simulink model "SensorTuner"  (R2024a)
settings: Solver=FixedStepAuto  StartTime=0.0  StopTime=3980  FixedStep=0.02  MinStep=0.1  RelTol=1e-3
values from neighbouring files (symbols this model uses):
  f = 0    [avg_error_f.m]
undefined symbols (not defined in the file or in its folder): dt, tau
settings Model: Creator=Pedro  LastModifiedBy=Pedro

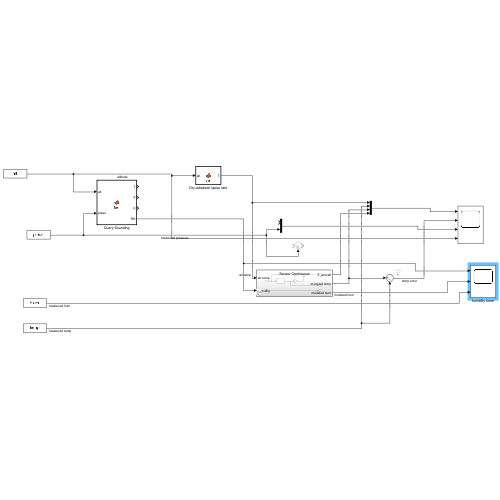
[thumbnail: Simulink's stored preview of the top-level diagram]
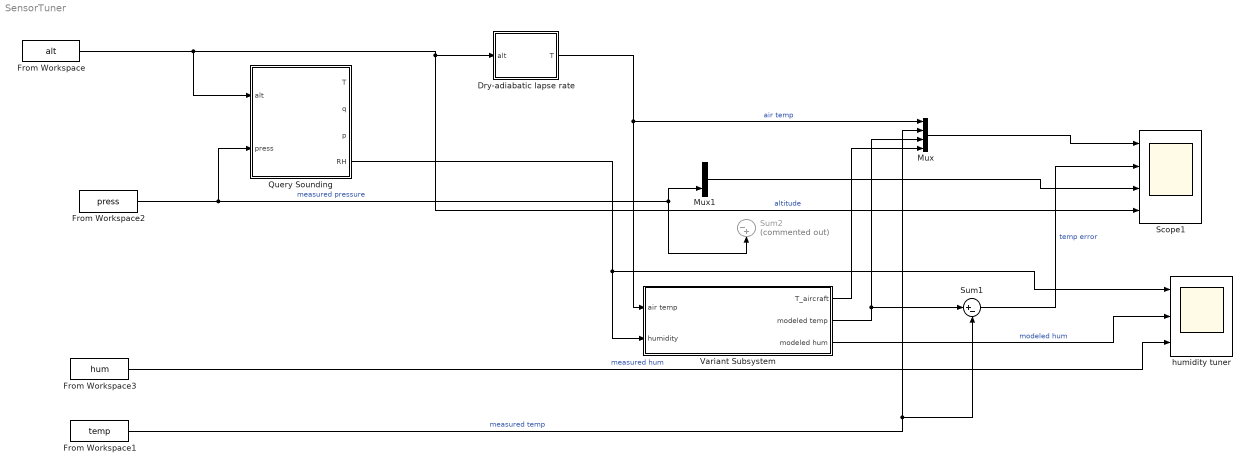
== system SensorTuner ==
  Dry-adiabatic lapse rate : MATLAB Function  TreatAsAtomicUnit=on
  From Workspace : FromWorkspace  VariableName=alt  OutputAfterFinalValue=Setting to zero
  From Workspace1 : FromWorkspace  VariableName=temp
  From Workspace2 : FromWorkspace  VariableName=press
  From Workspace3 : FromWorkspace  VariableName=hum
  Mux : Mux
  Mux1 : Mux  Inputs=2
  Query Sounding : MATLAB Function  TreatAsAtomicUnit=on
  Scope1 : Scope  NumInputPorts=4
  Sum1 : Sum  Inputs=|+-
  Sum2 : Sum  Commented=on  Inputs=|-+
  Variant Subsystem : Subsystem  Variant=on
  humidity tuner : Scope  NumInputPorts=3
  wires:
  Dry-adiabatic lapse rate/1(T) -> Variant Subsystem/1(air temp), Mux/1  "air temp"
  From Workspace/1 -> Query Sounding/1(alt), Dry-adiabatic lapse rate/1(alt), Scope1/4  "altitude"
  Mux/1 -> Scope1/1
  Sum1/1 -> Scope1/2  "temp error"
  From Workspace2/1 -> Query Sounding/2(press), Mux1/2, Sum2/2  "measured pressure"
  Mux1/1 -> Scope1/3
  From Workspace1/1 -> Sum1/2, Mux/2  "measured temp"
  Variant Subsystem/1(T_aircraft) -> Mux/4
  Variant Subsystem/2(modeled temp) -> Mux/3, Sum1/1
  Query Sounding/4(RH) -> humidity tuner/1, Variant Subsystem/2(humidity)
  Variant Subsystem/3(modeled hum) -> humidity tuner/2  "modeled hum"
  From Workspace3/1 -> humidity tuner/3  "measured hum"

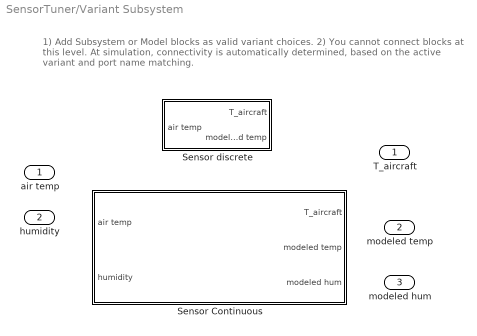
== system SensorTuner/Variant Subsystem ==
  note: 1) Add Subsystem or Model blocks as valid variant choices.
      | 2) You cannot connect blocks at this level. At simulation, connectivity is automatically
      | determined, based on the active variant and port name matching.
  air temp : Inport
  humidity : Inport  Port=2
  Sensor Continuous : Subsystem  VariantControl=true
  Sensor discrete : Subsystem  VariantControl=false
  T_aircraft : Outport
  modeled temp : Outport  Port=2
  modeled hum : Outport  Port=3

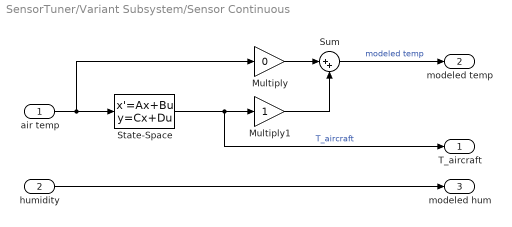
== system SensorTuner/Variant Subsystem/Sensor Continuous ==
  air temp : Inport
  humidity : Inport  Port=2
  Multiply : Gain  Gain=0
  Multiply1 : Gain
  State-Space : StateSpace  A=-(1/182.2415)  B=1/182.2415  D=0  InitialCondition=291.1304
  Sum : Sum  Inputs=|++
  T_aircraft : Outport
  modeled temp : Outport  Port=2
  modeled hum : Outport  Port=3
  wires:
  air temp/1 -> Multiply/1, State-Space/1
  State-Space/1 -> T_aircraft/1, Multiply1/1  "T_aircraft"
  Multiply/1 -> Sum/1
  Multiply1/1 -> Sum/2
  Sum/1 -> modeled temp/1  "modeled temp"
  humidity/1 -> modeled hum/1

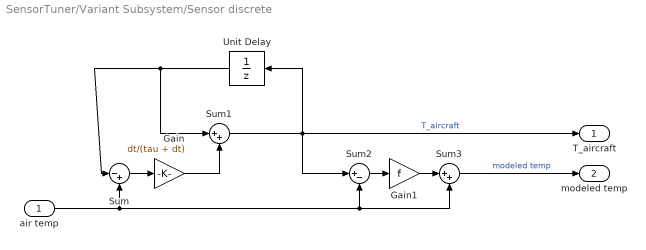
== system SensorTuner/Variant Subsystem/Sensor discrete ==
  air temp : Inport
  Gain : Gain  Gain=dt/(tau + dt)
  Gain1 : Gain  Gain=f
  Sum : Sum  Inputs=|-+
  Sum1 : Sum  Inputs=|++
  Sum2 : Sum  Inputs=|+-
  Sum3 : Sum  Inputs=|++
  Unit Delay : UnitDelay  InitialCondition=292.130400000000  SampleTime=-1  HasFrameUpgradeWarning=on
  T_aircraft : Outport
  modeled temp : Outport  Port=2
  wires:
  Unit Delay/1 -> Sum1/1, Sum/1
  air temp/1 -> Sum3/2, Sum2/2, Sum/2
  Sum/1 -> Gain/1
  Gain/1 -> Sum1/2
  Sum1/1 -> Unit Delay/1, T_aircraft/1, Sum2/1  "T_aircraft"
  Sum2/1 -> Gain1/1
  Gain1/1 -> Sum3/1
  Sum3/1 -> modeled temp/1  "modeled temp"

== matlab function SensorTuner/Dry-adiabatic lapse rate ==
  data: alt input; T output
function T = fcn(alt)

T = 300.9147 - 9.8 * (alt - 385)/1000;

== matlab function SensorTuner/Query Sounding ==
  data: alt input; press input; T output double size=1; q output double size=1; p output double size=1; sounding_buses parameter; RH output double size=1
function [T,q,p,RH] = fcn(alt,press,sounding_buses)


    T = 0.0;
    q = 0.0;
    p = 0.0;
    RH = 0.0;
    % Round aircraft height to nearest integer
    alt = round(alt);
    alt_top = alt + 0.01;
    alt_bottom = alt - 0.01;

    % Round pressure to nearest integer
    press = round(press);
    press_top = press + 0.5;
    press_bottom = press - 0.5;
    
    numLevels = sounding_buses.numLevels;
    logical_mask_press = false(numLevels,1);
    logical_mask = false(numLevels,1);
    used_soundings = false(1,1);

    % Initialize logical mask (1 if aircraft height is in sounding data, 0 otherwise)
    logical_mask = (sounding_buses.REPGPH <= alt_top & sounding_buses.REPGPH >= alt_bottom);
    logical_mask_press = (sounding_buses.PRESS <= press_top*100 & sounding_buses.PRESS >= press_bottom*100);
    % Check if no soundings contains the aircraft height
    if ~any(logical_mask)
        warning off backtrace
        warning('Aircraft height is not in sounding data');
        warning on backtrace
        return;
    end
    p = sounding_buses.PRESS(logical_mask);
    T = sounding_buses.TEMP(logical_mask);
    vap_press = sounding_buses.VAPPRESS(logical_mask);
    RH = sounding_buses.REPRH(logical_mask);

    % Compute the mixing ratio and specific humidity
    r = 0.622 * vap_press/(p - vap_press); % mixing ratio (kg water/kg dry air)
    q = r/(1 + r); % specific humidity (kg water/kg moist air)
    
    p = p(1,1)/100;
    T = T(1,1);
    q = q(1,1);

    % % Compute saturation vapor pressure (August-Roche-Magnus)
    % esat = 6.1094*exp(17.675*(T-273.15) / T - 273.15 + 243.04);
    % esat = esat(1,1);
    % RH = vap_press/esat;
    RH = RH(1,1);
end
